simulink model "readacc_final_3"  (R2017b)
settings: Solver=VariableStepAuto  StartTime=0.0  StopTime=15  RelTol=1e-3
libraries: dspstat3 x6, dspswit3 x5, instrumentlib x1
settings Model: NumberOfSteps=50  Creator=jmd  LastModifiedBy=jmd

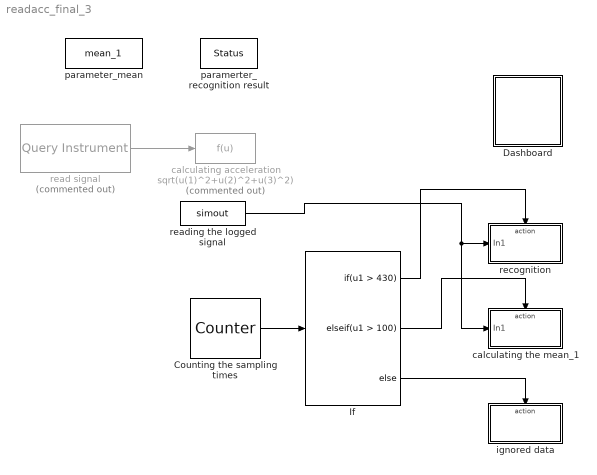
== system readacc_final_3 ==
  Counting the sampling times : dspswit3/Counter  Direction=Up  CountEvent=Free running  CounterSize=32 bits  MaxCount=255  InitialCount=0  Output=Count  HitValue=32  ResetInput=off  SamplesPerFrame=1  Ts=0.003  CntDtype=double  HitDtype=Logical
  Dashboard : Subsystem
  If : If  IfExpression=u1 > 430  ElseIfExpressions=u1 > 100
  calculating acceleration : Fcn  Commented=on  Expr=sqrt(u(1)^2+u(2)^2+u(3)^2)
  calculating the mean_1 : Subsystem  TreatAsAtomicUnit=on
  ignored data : Subsystem  TreatAsAtomicUnit=on
  paramerter_recognition result : DataStoreMemory  DataStoreName=Status  ReadBeforeWriteMsg=warning  WriteAfterWriteMsg=warning  WriteAfterReadMsg=warning  ShowAdditionalParam=off  OutDataTypeStr=double
  parameter_mean : DataStoreMemory  DataStoreName=mean_1  ReadBeforeWriteMsg=warning  WriteAfterWriteMsg=warning  WriteAfterReadMsg=warning  ShowAdditionalParam=off  OutDataTypeStr=double
  read signal : instrumentlib/Query Instrument  Commented=on  sampleTime=0.003  isWorkspaceObject=off  timeout=10  inputBufferSize=512  protocol=Serial  serialPort=COM1  baudRate=9600  gpibVendor=Agilent Technologies  boardIndex=0  primaryAddress=1  secondaryAddress=0  visaVendor=Agilent  visaSerialPort=0  chassisIndex=0  logicalAddress=0  tcpRemoteHost='127.0.0.1'  tcpRemotePort=4500  udpRemoteHost='127.0.0.1'  udpRemotePort=9090  visaTCPBoardIndex=0  visaTCPRemoteHost='127.0.0.1'  usbBoardIndex=0  usbManufID=0  usbModelCode=0  usbSerialNumber=0  initAction=None  initCommand='DATA:SOURCE CH1'  initFunction=get  queryCommand=''  responseFormat=Binary  asciiFormatting='%d,'  precision=8-bit integer  byteOrder=Little endian  valuesToRead=1  removeBytes=off  afterOutputAction=Repeat query for new data  enableFrames=on  frameSize=3
      settings: SourceProductName=Instrument Control Toolbox  SourceProductBaseCode=IC
  reading the logged signal : FromWorkspace  VariableName=simout  SampleTime=0.003
  recognition : Subsystem  TreatAsAtomicUnit=on
  wires:
  Counting the sampling times/1 -> If/1
  If/2 -> calculating the mean_1/Action
  If/3 -> ignored data/Action
  If/1 -> recognition/Action
  reading the logged signal/1 -> calculating the mean_1/1(In1), recognition/1(In1)
  read signal/1 -> calculating acceleration/1

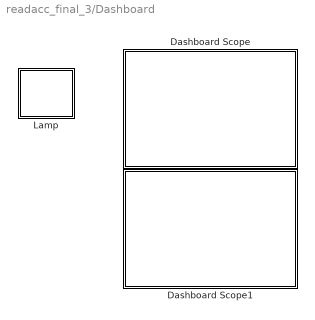
== system readacc_final_3/Dashboard ==
  Dashboard Scope : Subsystem  DialogController=hmiCreateDDGDialog  IsWebBlock=on  mask(MWDashboardBlock){webBlockId=a5a47974-a6a8-402f-a5cc-19f843840e52, webBlockType=sdiscope, ShowInitialText=on, HMISrcModelName=readacc_final_3}
      mask prompts: webBlockId "WebBlock Id"; webBlockType "WebBlock Type"; HMISrcModelName "Source Model"
      mask help: SimulinkHMI:dialogs:HMIScopeDialogDesc
      mask Help: helpview([docroot '/mapfiles/simulink.map'], 'hmi_scope')
      mask Display:
      | if strcmp(get_param(bdroot(gcb),'BlockDiagramType'), 'library')
      |     image([(matlabroot) '/toolbox/simulink/hmi/icons/DashboardScope.png']);
      | end
  Dashboard Scope1 : Subsystem  DialogController=hmiCreateDDGDialog  IsWebBlock=on  mask(MWDashboardBlock){webBlockId=b633f488-e0ae-4f95-8e06-777203ab0e40, webBlockType=sdiscope, ShowInitialText=on, HMISrcModelName=readacc_final_3}
      mask prompts: webBlockId "WebBlock Id"; webBlockType "WebBlock Type"; HMISrcModelName "Source Model"
      mask help: SimulinkHMI:dialogs:HMIScopeDialogDesc
      mask Help: helpview([docroot '/mapfiles/simulink.map'], 'hmi_scope')
      mask Display:
      | if strcmp(get_param(bdroot(gcb),'BlockDiagramType'), 'library')
      |     image([(matlabroot) '/toolbox/simulink/hmi/icons/DashboardScope.png']);
      | end
  Lamp : Subsystem  DialogController=hmiCreateDDGDialog  IsWebBlock=on  mask(MWDashboardBlock){webBlockId=bd819326-cf22-49c1-a3b0-f178f5fc1bdc, webBlockType=lamp, ShowInLibBrowser=on, ShowInitialText=on, HMISrcModelName=readacc_final_3}
      mask prompts: webBlockType "WebBlock Type"; HMISrcModelName "Source Model"
      mask help: SimulinkHMI:dialogs:LampDialogDesc
      mask Help: helpview([docroot '/mapfiles/simulink.map'], 'hmi_lamp')
      mask Display:
      | if strcmp(get_param(bdroot(gcb),'BlockDiagramType'), 'library')
      |     image([(matlabroot) '/toolbox/simulink/hmi/icons/Lamp.png']);
      | end

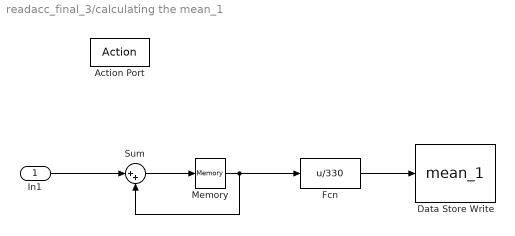
== system readacc_final_3/calculating the mean_1 ==
  In1 : Inport
  Action Port : ActionPort  ActionType=elseif
  Data Store Write : DataStoreWrite  DataStoreName=mean_1
  Fcn : Fcn  Expr=u/330
  Memory : Memory  InheritSampleTime=on
  Sum : Sum  Inputs=|++
  wires:
  In1/1 -> Sum/1
  Sum/1 -> Memory/1
  Fcn/1 -> Data Store Write/1
  Memory/1 -> Fcn/1, Sum/2

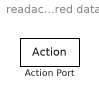
== system readacc_final_3/ignored data ==
  Action Port : ActionPort  ActionType=else

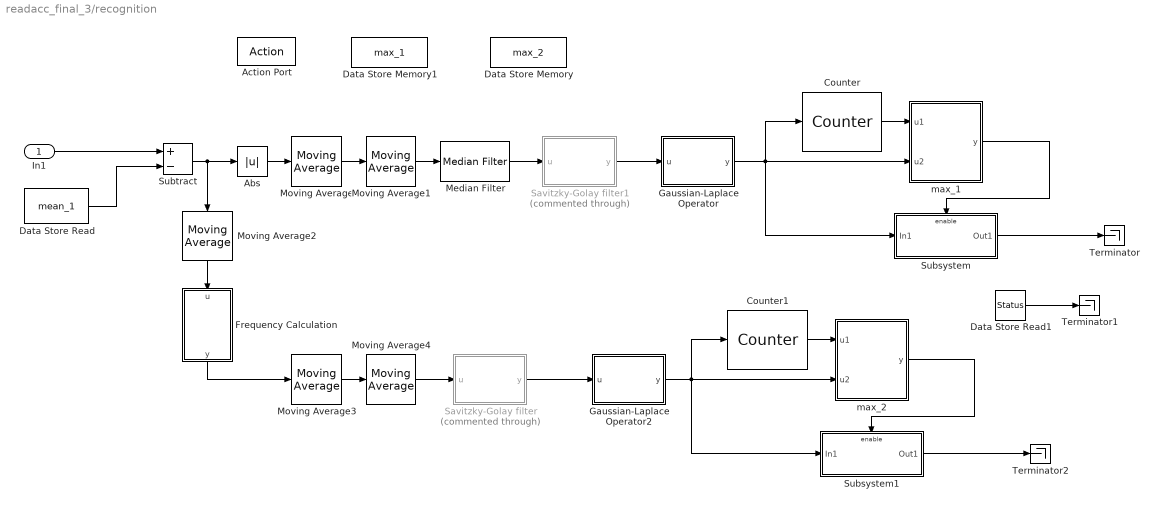
== system readacc_final_3/recognition ==
  In1 : Inport
  Action Port : ActionPort  InitializeStates=reset  ActionType=then
  Abs : Abs
  Counter : dspswit3/Counter  Direction=Up  CountEvent=Non-zero sample  CounterSize=16 bits  MaxCount=255  InitialCount=0  Output=Count  HitValue=32  ResetInput=off  SamplesPerFrame=1  Ts=1  CntDtype=double  HitDtype=Logical
  Counter1 : dspswit3/Counter  Direction=Up  CountEvent=Non-zero sample  CounterSize=16 bits  MaxCount=255  InitialCount=0  Output=Count  HitValue=32  ResetInput=off  SamplesPerFrame=1  Ts=1  CntDtype=double  HitDtype=Logical
  Data Store Memory : DataStoreMemory  DataStoreName=max_2  ReadBeforeWriteMsg=warning  WriteAfterWriteMsg=warning  WriteAfterReadMsg=warning  ShowAdditionalParam=off  OutDataTypeStr=double
  Data Store Memory1 : DataStoreMemory  DataStoreName=max_1  ReadBeforeWriteMsg=warning  WriteAfterWriteMsg=warning  WriteAfterReadMsg=warning  InitialValue=0.1  ShowAdditionalParam=off  OutDataTypeStr=double
  Data Store Read : DataStoreRead  DataStoreName=mean_1
  Data Store Read1 : DataStoreRead  DataStoreName=Status
  Frequency Calculation : MATLAB Function  TreatAsAtomicUnit=on
  Gaussian-Laplace Operator : MATLAB Function  TreatAsAtomicUnit=on
  Gaussian-Laplace Operator2 : MATLAB Function  TreatAsAtomicUnit=on
  Median Filter : dspstat3/Median Filter  WindowLength=20  SimulateUsing=Interpreted execution
      settings: SourceProductName=DSP System Toolbox  SourceProductBaseCode=DS
  Moving Average : dspstat3/Moving Average  Method=Sliding window  SpecifyWindowLength=on  WindowLength=137  ForgettingFactor=0.9  SimulateUsing=Code generation
  Moving Average1 : dspstat3/Moving Average  Method=Sliding window  SpecifyWindowLength=on  WindowLength=139  ForgettingFactor=0.9  SimulateUsing=Code generation
  Moving Average2 : dspstat3/Moving Average  Method=Sliding window  SpecifyWindowLength=on  WindowLength=3  ForgettingFactor=0.9  SimulateUsing=Code generation
  Moving Average3 : dspstat3/Moving Average  Method=Sliding window  SpecifyWindowLength=on  WindowLength=127  ForgettingFactor=0.9  SimulateUsing=Code generation
  Moving Average4 : dspstat3/Moving Average  Method=Sliding window  SpecifyWindowLength=on  WindowLength=131  ForgettingFactor=0.9  SimulateUsing=Code generation
  Savitzky-Golay filter : MATLAB Function  Commented=through  TreatAsAtomicUnit=on
  Savitzky-Golay filter1 : MATLAB Function  Commented=through  TreatAsAtomicUnit=on
  Subsystem : Subsystem
  Subsystem1 : Subsystem
  Subtract : Sum  Inputs=+-
  Terminator : Terminator
  Terminator1 : Terminator
  Terminator2 : Terminator
  max_1 : MATLAB Function  TreatAsAtomicUnit=on
  max_2 : MATLAB Function  TreatAsAtomicUnit=on
  wires:
  Subtract/1 -> Moving Average2/1, Abs/1
  Data Store Read/1 -> Subtract/2
  Moving Average/1 -> Moving Average1/1
  In1/1 -> Subtract/1
  Abs/1 -> Moving Average/1
  Median Filter/1 -> Savitzky-Golay filter1/1(u)
  Gaussian-Laplace Operator/1(y) -> max_1/2(u2), Subsystem/1(In1), Counter/1
  Counter/1 -> max_1/1(u1)
  Moving Average1/1 -> Median Filter/1
  max_1/1(y) -> Subsystem/Enable
  Subsystem/1(Out1) -> Terminator/1
  Moving Average2/1 -> Frequency Calculation/1(u)
  Frequency Calculation/1(y) -> Moving Average3/1
  Moving Average3/1 -> Moving Average4/1
  max_2/1(y) -> Subsystem1/Enable
  Gaussian-Laplace Operator2/1(y) -> Subsystem1/1(In1), max_2/2(u2), Counter1/1
  Counter1/1 -> max_2/1(u1)
  Subsystem1/1(Out1) -> Terminator2/1
  Moving Average4/1 -> Savitzky-Golay filter/1(u)
  Data Store Read1/1 -> Terminator1/1
  Savitzky-Golay filter/1(y) -> Gaussian-Laplace Operator2/1(u)
  Savitzky-Golay filter1/1(y) -> Gaussian-Laplace Operator/1(u)

== system readacc_final_3/Dashboard/Dashboard Scope ==

== system readacc_final_3/Dashboard/Dashboard Scope1 ==

== system readacc_final_3/Dashboard/Lamp ==

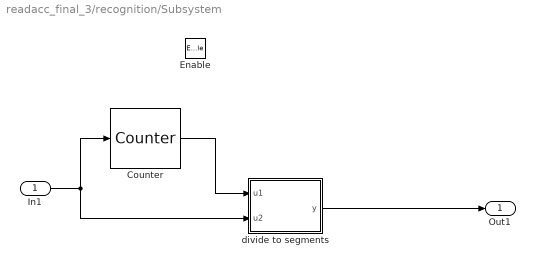
== system readacc_final_3/recognition/Subsystem ==
  In1 : Inport
  Enable : EnablePort
  Counter : dspswit3/Counter  Direction=Up  CountEvent=Non-zero sample  CounterSize=User defined  MaxCount=250  InitialCount=1  Output=Count  HitValue=32  ResetInput=off  SamplesPerFrame=1  Ts=1  CntDtype=double  HitDtype=Logical
  divide to segments : MATLAB Function  TreatAsAtomicUnit=on
  Out1 : Outport
  wires:
  In1/1 -> divide to segments/2(u2), Counter/1
  Counter/1 -> divide to segments/1(u1)
  divide to segments/1(y) -> Out1/1

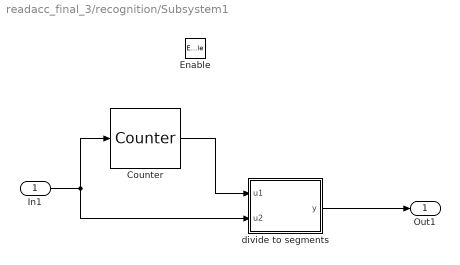
== system readacc_final_3/recognition/Subsystem1 ==
  In1 : Inport
  Enable : EnablePort
  Counter : dspswit3/Counter  Direction=Up  CountEvent=Non-zero sample  CounterSize=User defined  MaxCount=250  InitialCount=1  Output=Count  HitValue=32  ResetInput=off  SamplesPerFrame=1  Ts=1  CntDtype=double  HitDtype=Logical
  divide to segments : MATLAB Function  TreatAsAtomicUnit=on
  Out1 : Outport
  wires:
  In1/1 -> divide to segments/2(u2), Counter/1
  Counter/1 -> divide to segments/1(u1)
  divide to segments/1(y) -> Out1/1

== matlab function readacc_final_3/recognition/Gaussian-Laplace Operator ==
  data: u input; y output
function y = fcn(u)

persistent len_1 counter_1 ;
if isempty(len_1)
    len_1 = zeros(1,100);
    counter_1 = 0;
end
counter_1 = counter_1 +1;
len_1 = [len_1(2:100), u];
if counter_1 >361
    y = (3*u - 2*len_1(50)-len_1(1))^2;
else
    y = 0;
end

== matlab function readacc_final_3/recognition/max_1 ==
  data: u1 input; u2 input; y output; max_1 data_store_memory
function y = fcn(u1, u2)

global max_1
if u1<600
    if u2>max_1
        max_1 = u2;
    end
    y = 0;
else
    y = 1;
end

== matlab function readacc_final_3/recognition/Frequency Calculation ==
  data: u input; y output
function y = fcn(u)

persistent sign counter c d timepoint fre;

if isempty(sign)
    sign = 1;
    counter = 0;
    c = 0;
    d = [u u u];
    timepoint = zeros(1,3);
    fre = 0;
end
d = [d(2:3) u];
if (d(2)*sign) <= 0 && (d(3)*sign) <= 0
    sign = -sign;
    c = c +1;
    timepoint(c) = counter-1 + d(1)/(d(1)-d(2));
    if c == 3
        fre = 330/(timepoint(3)-timepoint(1));
        c = 1;
        timepoint(1) = timepoint(3);   
    end
end
u2 = u;
counter = counter + 1;
y = fre;

== matlab function readacc_final_3/recognition/Subsystem/divide to segments ==
  data: u1 input; y output; u2 input; max_1 data_store_memory; Status data_store_memory
function y = fcn(u1,u2)

global max_1 Status

persistent local_max
if isempty(local_max)
    local_max=[0.1 0.1];
end
if u1==250
    local_max(1) = local_max(2);
    local_max(2) = 0;
end 

if u2>local_max(2)
    local_max(2) = u2;
end

if (4*max_1)<local_max(1)
    y = 20;
    Status = 1;
elseif local_max(1)>max_1
    max_1 = 0.5*(max_1+(1));
    y=5;
else
    y=5;
end

== matlab function readacc_final_3/recognition/Gaussian-Laplace Operator2 ==
  data: u input; y output
function y = fcn(u)

persistent len_1 counter_1 ;
if isempty(len_1)
    len_1 = zeros(1,100);
    counter_1 = 0;
end
counter_1 = counter_1 +1;
len_1 = [len_1(2:100), u];
if counter_1 >361
    y = (3*u - 2*len_1(50)-len_1(1))^2;
else
    y = 0;
end

== matlab function readacc_final_3/recognition/max_2 ==
  data: u1 input; u2 input; y output; max_2 data_store_memory
function y = fcn(u1, u2)

global max_2
if u1<600
    if u2>max_2
        max_2 = u2;
    end
    y = 0;
else
    y = 1;
end

== matlab function readacc_final_3/recognition/Subsystem1/divide to segments ==
  data: u1 input; y output; u2 input; max_2 data_store_memory; Status data_store_memory
function y = fcn(u1,u2)

global max_2 Status

persistent local_max
if isempty(local_max)
    local_max=[0.1 0.1];
end
if u1==250
    local_max(1) = local_max(2);
    local_max(2) = 0;
end 

if u2>local_max(2)
    local_max(2) = u2;
end

if (4*max_2)<local_max(1)
    y = 20;
    Status = 1;
elseif local_max(1)>max_2
    max_2 = 0.5*(max_2+(1));
    y=5;
else
    y=5;
end

== matlab function readacc_final_3/recognition/Savitzky-Golay filter ==
  data: u input; y output
function y = fcn(u)

persistent x;
if isempty(x)
    x=zeros(1,100);
end
x=[x(2:100),u];
m=5;
n=length(x);
  a=x;
for k=1: m
 b(1) = (69*a(1) +4*(a(2) +a(4)) -6*a(3) -a(5)) /70;
 b(2) = (2* (a(1) +a(5)) +27*a(2) +12*a(3) -8*a(4)) /35;
 for j=3:n-2
   b (j) = (-3*(a(j-2) +a(j+2)) +12*(a(j-1) +a(j+1)) +17*a(j)) /35;
 end
 b (n-1) = (2*(a(n) +a(n-4)) +27*a(n-1) +12*a(n-2) -8*a(n-3)) /35;
 b (n) = (69*a(n) +4* (a(n-1) +a(n-3)) -6*a(n-2) -a(n-4)) /70;
 a=b;
end
y =a;

== matlab function readacc_final_3/recognition/Savitzky-Golay filter1 ==
  data: u input; y output
function y = fcn(u)

persistent x;
if isempty(x)
    x=zeros(1,100);
end
x=[x(2:100),u];
m=5;
n=length(x);
  a=x;
for k=1: m
 b(1) = (69*a(1) +4*(a(2) +a(4)) -6*a(3) -a(5)) /70;
 b(2) = (2* (a(1) +a(5)) +27*a(2) +12*a(3) -8*a(4)) /35;
 for j=3:n-2
   b (j) = (-3*(a(j-2) +a(j+2)) +12*(a(j-1) +a(j+1)) +17*a(j)) /35;
 end
 b (n-1) = (2*(a(n) +a(n-4)) +27*a(n-1) +12*a(n-2) -8*a(n-3)) /35;
 b (n) = (69*a(n) +4* (a(n-1) +a(n-3)) -6*a(n-2) -a(n-4)) /70;
 a=b;
end
y =a;
